simulink model "prelab2_simulink"  (R2017a)
settings: Solver=ode45  StartTime=0.0  StopTime=3.0  MaxStep=.001  RelTol=1e-3
settings Model: Creator=kg3  LastModifiedBy=kg3

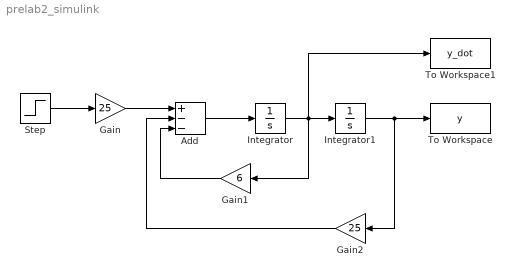
== system prelab2_simulink ==
  Add : Sum  Inputs=+--
  Gain : Gain  Gain=25
  Gain1 : Gain  Gain=6
  Gain2 : Gain  Gain=25
  Integrator : Integrator
  Integrator1 : Integrator
  Step : Step  Time=0  SampleTime=0
  To Workspace : ToWorkspace  VariableName=y  SampleTime=-1
  To Workspace1 : ToWorkspace  VariableName=y_dot  SampleTime=-1
  wires:
  Step/1 -> Gain/1
  Integrator/1 -> To Workspace1/1, Gain1/1, Integrator1/1
  Integrator1/1 -> Gain2/1, To Workspace/1
  Add/1 -> Integrator/1
  Gain/1 -> Add/1
  Gain1/1 -> Add/3
  Gain2/1 -> Add/2
